simulink model "turbulance"  (R2016b)
settings: Solver=VariableStepAuto  StartTime=0.0  StopTime=10.0  RelTol=1e-3
libraries: simulink x1
settings Model: Creator=charAn  LastModifiedBy=charAn

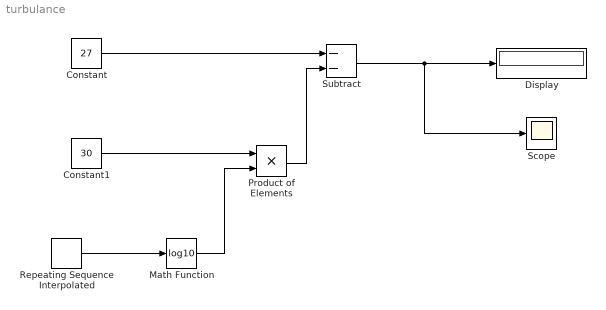
== system turbulance ==
  Constant : Constant  Value=27
  Constant1 : Constant  Value=30
  Display : Display
  Math Function : Math  Operator=log10  SaturateOnIntegerOverflow=on
  Product of Elements : Product
  Repeating Sequence Interpolated : simulink/Sources/Repeating Sequence Interpolated  OutValues=[0 5 10 15 20]  TimeValues=[0 5 10 15 20]  LookUpMeth=Interpolation-Use End Values  tsamp=0.01  OutMin=[]  OutMax=[]  OutDataTypeStr=double  OutputDataTypeScalingMode=double  OutDataType=fixdt(0,8)  OutScaling=2^-10
  Scope : Scope
  Subtract : Sum  Inputs=--
  wires:
  Constant/1 -> Subtract/1
  Constant1/1 -> Product of Elements/1
  Repeating Sequence Interpolated/1 -> Math Function/1
  Math Function/1 -> Product of Elements/2
  Product of Elements/1 -> Subtract/2
  Subtract/1 -> Scope/1, Display/1
